simulink model "DoubleTankSim_SlidingModeCtrl"  (R2025b)
settings: Solver=ode5  StartTime=0.0  StopTime=1500  FixedStep=Ts  RelTol=1e-3  EnableMultiTasking=on
values from neighbouring files (symbols this model uses):
  a_1 = 0.15025    [LabC.m]
  a_2 = 0.15615    [LabC.m]
  At = 33    [LabC.m]
  g = 981    [LabC.m]
  h_0 = 3.2    [LabC.m]
  k = 0.1    [LabC.m]
  lambda = 0.04    [LabC.m]
  phi = 0.1    [LabC.m]
  Q = [variance 0 0 ... (first row only)    [LabC.m]
  R = 1    [LabC.m]
  Ts = 0.02    [LabC.m]
  variance = 1e-5    (= 1e-05)    [LabC.m]
libraries: simulink x3
settings Model: Creator=kaspe  LastModifiedBy=kaspe
settings SolverCC: AutoInsertRateTranBlk=on

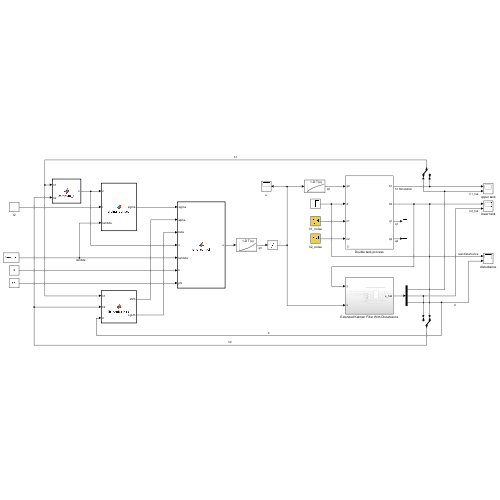
[thumbnail: Simulink's stored preview of the top-level diagram]
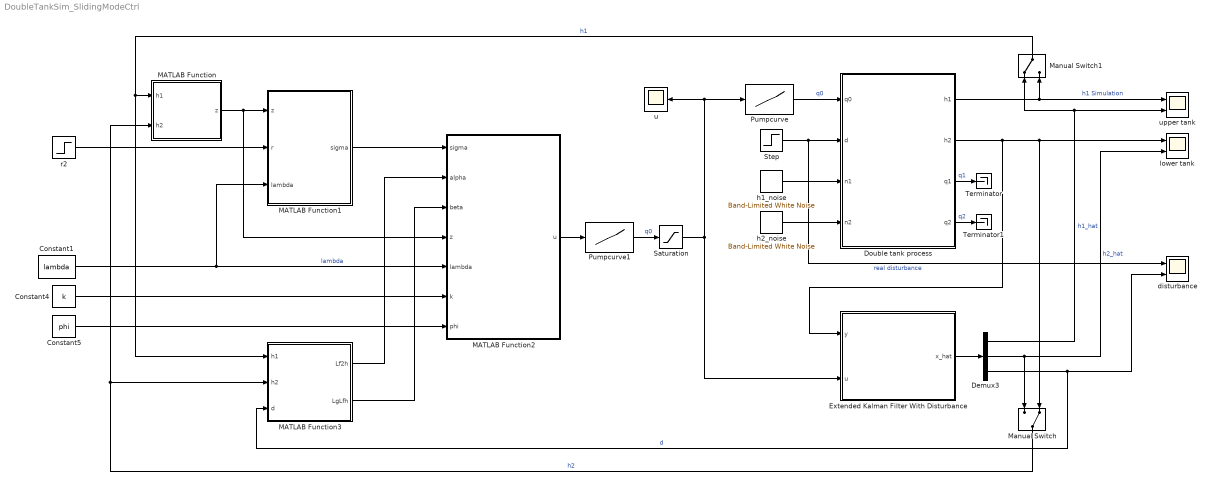
== system DoubleTankSim_SlidingModeCtrl ==
  Constant1 : Constant  Value=lambda
  Constant4 : Constant  Value=k
  Constant5 : Constant  Value=phi
  Demux3 : Demux  Outputs=3
  Double tank process : Subsystem  mask{At=33, a_1=0.16, a_2=0.15, hmax=15.5}
      mask prompts: At "Tank area (cm^2)"; a_1 "Upper tank opening area (cm^2)"; a_2 "Lower tank opening area (cm^2)"; hmax "Tank height (cm)"
      mask help: Double tank process parameters
  Extended Kalman Filter With Disturbance : Subsystem
  MATLAB Function : MATLAB Function  TreatAsAtomicUnit=on
  MATLAB Function1 : MATLAB Function  TreatAsAtomicUnit=on
  MATLAB Function2 : MATLAB Function  TreatAsAtomicUnit=on
  MATLAB Function3 : MATLAB Function  TreatAsAtomicUnit=on
  Manual Switch : ManualSwitch  CurrentSetting=0
  Manual Switch1 : ManualSwitch
  Pumpcurve : Lookup_n-D  NumberOfTableDimensions=1  BreakpointsForDimension1=x  BreakpointsForDimension2=[1:3]  Table=y  RndMeth=Simplest  mask{x=[0.5,1,1.5,2,2.5,3,3.5,5,8,10], y=[16.47,20.75,24.52,27.63,30.06,32.49,34.80,40.28,48.24,52.43]}
      mask prompts: x "Values on x-axis"; y "Values on y-axis"
  Pumpcurve1 : Lookup_n-D  NumberOfTableDimensions=1  BreakpointsForDimension1=x  BreakpointsForDimension2=[1:3]  Table=y  RndMeth=Simplest  mask{x=[16.47,20.75,24.52,27.63,30.06,32.49,34.80,40.28,48.24,52.43], y=[0.5,1,1.5,2,2.5,3,3.5,5,8,10]}
      mask prompts: x "Values on x-axis"; y "Values on y-axis"
  Saturation : Saturate  UpperLimit=10  LowerLimit=0
  Step : Step  Time=900  After=0.05  SampleTime=0
  Terminator : Terminator
  Terminator1 : Terminator
  disturbance : Scope  NumInputPorts=2
      settings: ActiveDisplayYMinimum=-0.062238391990191946  ActiveDisplayYMaximum=0.088631912963099843  DataLoggingVariableName=ScopeData2
  h1_noise : simulink/Sources/Band-Limited White Noise  Cov=[variance]  Ts=Ts  seed=[23342]
  h2_noise : simulink/Sources/Band-Limited White Noise  Cov=[variance]  Ts=Ts  seed=[23341]
  lower tank : Scope  NumInputPorts=2
      settings: ActiveDisplayYMinimum=-1.8792470771326775  ActiveDisplayYMaximum=9.9236230933601934
  r2 : Step  Time=500  Before=8  After=12  SampleTime=0
  u : Scope
      settings: ActiveDisplayYMinimum=0.83678012051645867  ActiveDisplayYMaximum=1.7740163831360298  DataLoggingVariableName=ScopeData3
  upper tank : Scope  NumInputPorts=2
      settings: ActiveDisplayYMinimum=-3.2062616403720225  ActiveDisplayYMaximum=23.260867883812139
  wires:
  Pumpcurve/1 -> Double tank process/1(q0)  "q0"
  Double tank process/1(h1) -> Manual Switch1/2, upper tank/1  "h1 Simulation"
  Step/1 -> Double tank process/2(d), disturbance/1  "real disturbance"
  h1_noise/1 -> Double tank process/3(n1)
  h2_noise/1 -> Double tank process/4(n2)
  Demux3/1 -> Manual Switch1/1, upper tank/2  "h1_hat"
  Double tank process/2(h2) -> Extended Kalman Filter With Disturbance/1(y), Manual Switch/2, lower tank/1
  Demux3/2 -> lower tank/2, Manual Switch/1  "h2_hat"
  Demux3/3 -> MATLAB Function3/3(d), disturbance/2  "d"
  Saturation/1 -> Extended Kalman Filter With Disturbance/2(u), u/1, Pumpcurve/1
  Double tank process/3(q1) -> Terminator/1  "q1"
  Double tank process/4(q2) -> Terminator1/1  "q2"
  r2/1 -> MATLAB Function1/2(r)
  Extended Kalman Filter With Disturbance/1(x_hat) -> Demux3/1
  MATLAB Function/1(z) -> MATLAB Function1/1(z), MATLAB Function2/4(z)
  MATLAB Function2/1(u) -> Pumpcurve1/1
  MATLAB Function3/1(Lf2h) -> MATLAB Function2/2(alpha)
  MATLAB Function3/2(LgLfh) -> MATLAB Function2/3(beta)
  MATLAB Function1/1(sigma) -> MATLAB Function2/1(sigma)
  Constant5/1 -> MATLAB Function2/7(phi)
  Constant1/1 -> MATLAB Function2/5(lambda), MATLAB Function1/3(lambda)  "lambda"
  Constant4/1 -> MATLAB Function2/6(k)
  Manual Switch/1 -> MATLAB Function/2(h2), MATLAB Function3/2(h2)  "h2"
  Manual Switch1/1 -> MATLAB Function/1(h1), MATLAB Function3/1(h1)  "h1"
  Pumpcurve1/1 -> Saturation/1  "q0"

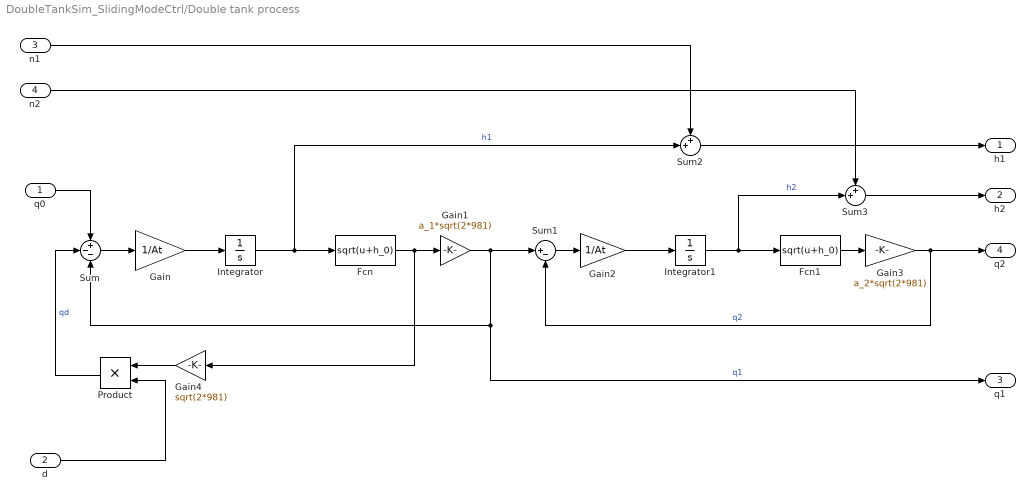
== system DoubleTankSim_SlidingModeCtrl/Double tank process ==
  q0 : Inport
  d : Inport  Port=2
  n1 : Inport  Port=3
  n2 : Inport  Port=4
  Fcn : Fcn  Expr=sqrt(u+h_0)
  Fcn1 : Fcn  Expr=sqrt(u+h_0)
  Gain : Gain  Gain=1/At
  Gain1 : Gain  Gain=a_1*sqrt(2*981)
  Gain2 : Gain  Gain=1/At
  Gain3 : Gain  Gain=a_2*sqrt(2*981)
  Gain4 : Gain  Gain=sqrt(2*981)
  Integrator : Integrator  LimitOutput=on  UpperSaturationLimit=hmax  LowerSaturationLimit=0
  Integrator1 : Integrator  LimitOutput=on  UpperSaturationLimit=hmax  LowerSaturationLimit=0
  Product : Product  RndMeth=Zero
  Sum : Sum  Inputs=+--
  Sum1 : Sum  Inputs=|+-
  Sum2 : Sum  Inputs=++|
  Sum3 : Sum  Inputs=++|
  h1 : Outport  VectorParamsAs1DForOutWhenUnconnected=off
  h2 : Outport  Port=2  VectorParamsAs1DForOutWhenUnconnected=off
  q1 : Outport  Port=3  VectorParamsAs1DForOutWhenUnconnected=off
  q2 : Outport  Port=4  VectorParamsAs1DForOutWhenUnconnected=off
  wires:
  Sum/1 -> Gain/1
  Gain/1 -> Integrator/1
  Fcn/1 -> Gain4/1, Gain1/1
  Gain1/1 -> Sum1/1, q1/1, Sum/3  "q1"
  Sum1/1 -> Gain2/1
  Gain2/1 -> Integrator1/1
  Fcn1/1 -> Gain3/1
  Gain3/1 -> Sum1/2, q2/1  "q2"
  q0/1 -> Sum/1
  Integrator/1 -> Sum2/2, Fcn/1  "h1"
  Product/1 -> Sum/2  "qd"
  Integrator1/1 -> Sum3/2, Fcn1/1  "h2"
  d/1 -> Product/2
  Sum2/1 -> h1/1
  n1/1 -> Sum2/1
  Sum3/1 -> h2/1
  n2/1 -> Sum3/1
  Gain4/1 -> Product/1

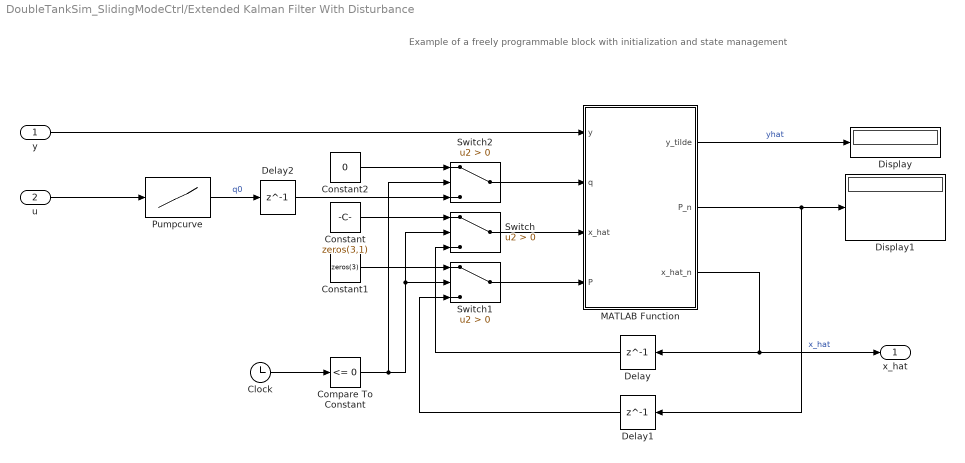
== system DoubleTankSim_SlidingModeCtrl/Extended Kalman Filter With Disturbance ==
  note: Example of a freely programmable block with initialization and state management
  y : Inport
  u : Inport  Port=2
  Clock : Clock
  Compare To Constant : simulink/Logic and Bit Operations/Compare To Constant  relop=<=  const=0  OutDataTypeStr=boolean
  Constant : Constant  Value=zeros(3,1)
  Constant1 : Constant  Value=zeros(3)
  Constant2 : Constant  Value=0
  Delay : Delay  DelayLength=1  InitialCondition=0
  Delay1 : Delay  DelayLength=1  InitialCondition=0
  Delay2 : Delay  DelayLength=1  InitialCondition=0
  Display : Display
  Display1 : Display
  MATLAB Function : MATLAB Function  TreatAsAtomicUnit=on
  Pumpcurve : Lookup_n-D  NumberOfTableDimensions=1  BreakpointsForDimension1=x  BreakpointsForDimension2=[1:3]  Table=y  RndMeth=Simplest  mask{x=[0.5,1,1.5,2,2.5,3,3.5,5,8,10], y=[16.47,20.75,24.52,27.63,30.06,32.49,34.80,40.28,48.24,52.43]}
      mask prompts: x "Values on x-axis"; y "Values on y-axis"
  Switch : Switch  Criteria=u2 > Threshold  SaturateOnIntegerOverflow=off  InputSameDT=off
  Switch1 : Switch  Criteria=u2 > Threshold  SaturateOnIntegerOverflow=off  InputSameDT=off
  Switch2 : Switch  Criteria=u2 > Threshold  SaturateOnIntegerOverflow=off  InputSameDT=off
  x_hat : Outport  PortDimensions=3
  wires:
  Delay/1 -> Switch/3
  Switch/1 -> MATLAB Function/3(x_hat)
  Constant1/1 -> Switch1/1
  Compare To Constant/1 -> Switch2/2, Switch/2, Switch1/2
  Constant/1 -> Switch/1
  MATLAB Function/1(y_tilde) -> Display/1  "yhat"
  MATLAB Function/2(P_n) -> Delay1/1, Display1/1
  Clock/1 -> Compare To Constant/1
  Switch1/1 -> MATLAB Function/4(P)
  y/1 -> MATLAB Function/1(y)
  Delay1/1 -> Switch1/3
  Switch2/1 -> MATLAB Function/2(q)
  Constant2/1 -> Switch2/1
  Delay2/1 -> Switch2/3
  Pumpcurve/1 -> Delay2/1  "q0"
  u/1 -> Pumpcurve/1
  MATLAB Function/3(x_hat_n) -> Delay/1, x_hat/1  "x_hat"

== matlab function DoubleTankSim_SlidingModeCtrl/MATLAB Function ==
  data: h1 input; z output; h2 input; h_0 parameter; a_1 parameter; a_2 parameter; At parameter; g parameter
function z = compute_z(h1, h2, h_0, a_1, a_2, At, g)
    Q1 = sqrt(2*g*(h1 + h_0));
    Q2 = sqrt(2*g*(h2 + h_0));

    z = [h2;                         % z₁ = h(x)
         (a_1*Q1 - a_2*Q2) / At];     % z₂ = Lf h(x) = ẋ₂
end

== matlab function DoubleTankSim_SlidingModeCtrl/MATLAB Function1 ==
  data: z input; sigma output; r input; lambda input
function sigma = sliding_surface(z, r, lambda)
    e  = z(1) - r;
    de = z(2);
    sigma = de + lambda*e;
end

== matlab function DoubleTankSim_SlidingModeCtrl/Extended Kalman Filter With Disturbance/MATLAB Function ==
  data: y input; q input; x_hat input; At parameter; a_1 parameter; a_2 parameter; h_0 parameter; y_tilde output; P input; P_n output; x_hat_n output; Q parameter; R parameter; g parameter; Ts parameter
function [y_tilde, P_n, x_hat_n] = fcn(y, q, x_hat, At, a_1, a_2, h_0, P, Q, R, g, Ts)

% Linearization
h_hat1 = x_hat(1);
h_hat2 = x_hat(2);
a_l = x_hat(3);

sqrt1 = sqrt(2*g*(max([h_hat1+h_0,0])));
sqrt2 = sqrt(2*g*(max([h_hat2+h_0,0])));

A = [-(a_1 + a_l)*g/At/sqrt1, 0,              -sqrt1/At;
     a_1*g/At/sqrt1,           -a_2*g/At/sqrt2, 0
     0,                       0,              0];

C = [0 1 0];

Ad = eye(size(A)) + Ts * A;

% Predict
x_hat_dot = [(q - (a_1 + a_l)*sqrt1)/At; 
             (a_1*sqrt1 - a_2*sqrt2)/At;
             0];
x_hat_n = x_hat + x_hat_dot .* Ts;
P_n = Ad * P * Ad' + Q;

% Update
y_tilde = y - C * x_hat_n;
S = C * P_n * C' + R;
K = P_n * C' * inv(S);
x_hat_n = x_hat_n + K * y_tilde;

P_n = (eye(size(A)) - K * C) * P_n;   
y_tilde = y - C * x_hat_n;

== matlab function DoubleTankSim_SlidingModeCtrl/MATLAB Function2 ==
  data: sigma input; u output size=1; alpha input; beta input; z input; lambda input; k input; phi input
function u = smc_control(sigma, alpha, beta,  ...
                          z, lambda, k, phi)

    % Virtual input (SMC law)
    v = lambda*z(2) - k*sat(sigma, phi);

    % Reverse feedback linearization
    u = (v - alpha) / beta;
end

function y = sat(x, phi)
    y = max(-1, min(1, x/phi));
end

== matlab function DoubleTankSim_SlidingModeCtrl/MATLAB Function3 ==
  data: h1 input; Lf2h output; h2 input; d input; LgLfh output; a_1 parameter; a_2 parameter; h_0 parameter; At parameter; g parameter
function [Lf2h, LgLfh] = lie_derivatives(h1, h2, d, a_1, a_2, h_0, At, g)
    Q1 = sqrt(2*g*(h1+h_0));
    Q2 = sqrt(2*g*(h2+h_0));

    f1 = (-(a_1 + d)*Q1) / At;   % no u term for Lie derivative
    f2 = (a_1*Q1 - a_2*Q2) / At;

    dF2_dx1 =  a_1*Q1 / (2*At*(h1+h_0));
    dF2_dx2 = -a_2*Q2 / (2*At*(h2+h_0));

    Lf2h  = dF2_dx1*f1 + dF2_dx2*f2;
    LgLfh = dF2_dx1 * (1/At);
end
